simulink model "FuzzySL"  (R2018b)
settings: Solver=VariableStepAuto  StartTime=0.0  StopTime=10.0  RelTol=1e-3
libraries: fuzblock x1
settings Model: Creator=student  LastModifiedBy=Harsh

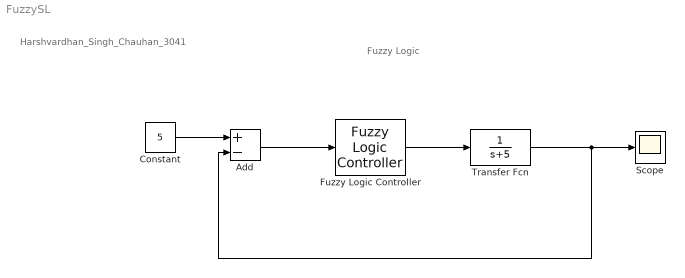
== system FuzzySL ==
  note: Fuzzy Logic
  note: Harshvardhan_Singh_Chauhan_3041
  Add : Sum  Inputs=+-
  Constant : Constant  Value=5
  Fuzzy Logic Controller : fuzblock/Fuzzy Logic  Controller  FIS='Fuzzy1.fis'  OutputSampleNumber=101  DataType=double  FuzzifiedInputs=off  RuleFiringStrengths=off  RuleOutputs=off  AggregatedOutputs=off  SimulateUsing=Interpreted execution  OutOfRangeInputValueMessage=warning  NoRuleFiredMessage=warning  EmptyOutputFuzzySetMessage=warning
  Scope : Scope
  Transfer Fcn : TransferFcn  Denominator=[1 5]
  wires:
  Constant/1 -> Add/1
  Add/1 -> Fuzzy Logic Controller/1
  Fuzzy Logic Controller/1 -> Transfer Fcn/1
  Transfer Fcn/1 -> Scope/1, Add/2
